simulink model "Controller_bis"  (R2019b)
settings: Solver=VariableStepAuto  StartTime=0.0  StopTime=10.0  RelTol=1e-3
undefined symbols (not defined in the file): B, b1, b2, C, D, gravity, K, KControl, l, q0
settings Model: Creator=ariannagasparri  LastModifiedBy=giga4
settings DebuggingCC: UnderSpecifiedDimensionMsg=warning

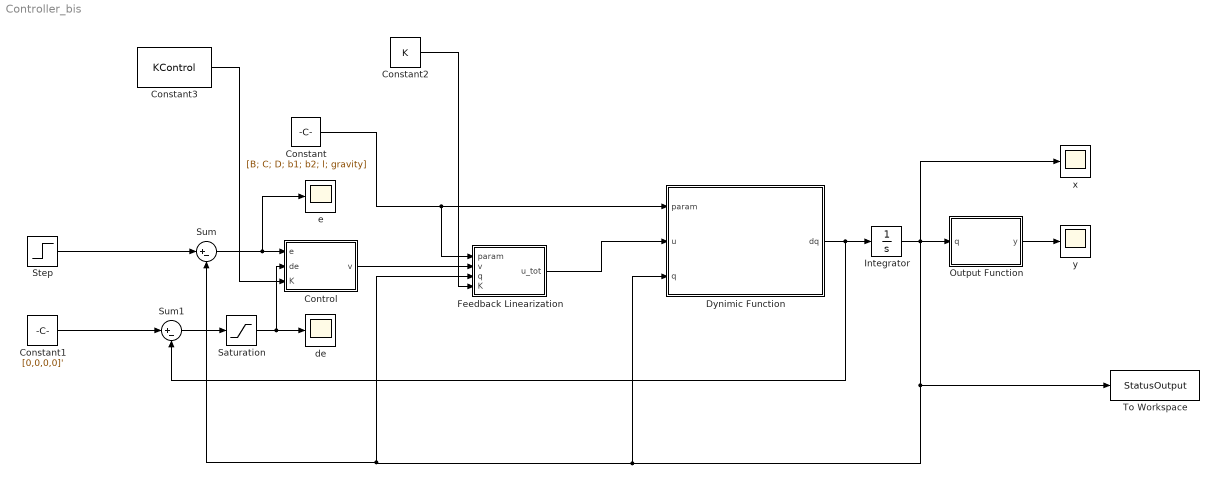
== system Controller_bis ==
  Constant : Constant  Value=[B; C; D; b1; b2; l; gravity]
  Constant1 : Constant  Value=[0,0,0,0]'
  Constant2 : Constant  Value=K
  Constant3 : Constant  Value=KControl
  Control : MATLAB Function  TreatAsAtomicUnit=on
  Dynimic Function : MATLAB Function  TreatAsAtomicUnit=on
  Feedback Linearization : MATLAB Function  TreatAsAtomicUnit=on
  Integrator : Integrator  InitialCondition=q0
  Output Function : MATLAB Function  TreatAsAtomicUnit=on
  Saturation : Saturate  UpperLimit=[10,10,10,10]'  LowerLimit=-[10,10,10,10]'
  Step : Step  After=[0,0,3,0]'  SampleTime=0
  Sum : Sum  Inputs=|+-
  Sum1 : Sum  Inputs=|+-
  To Workspace : ToWorkspace  VariableName=StatusOutput  SaveFormat=Timeseries  SampleTime=-1
  de : Scope
  e : Scope
  x : Scope
  y : Scope
  wires:
  Integrator/1 -> To Workspace/1, Dynimic Function/3(q), Sum/2, Feedback Linearization/3(q), x/1, Output Function/1(q)
  Constant/1 -> Feedback Linearization/1(param), Dynimic Function/1(param)
  Sum1/1 -> Saturation/1
  Dynimic Function/1(dq) -> Sum1/2, Integrator/1
  Sum/1 -> e/1, Control/1(e)
  Output Function/1(y) -> y/1
  Control/1(v) -> Feedback Linearization/2(v)
  Step/1 -> Sum/1
  Constant1/1 -> Sum1/1
  Feedback Linearization/1(u_tot) -> Dynimic Function/2(u)
  Saturation/1 -> Control/2(de), de/1
  Constant2/1 -> Feedback Linearization/4(K)
  Constant3/1 -> Control/3(K)

== matlab function Controller_bis/Feedback Linearization ==
  data: param input; v input; u_tot output; q input; K input
function u_tot = fcn(param, v, q, K)

u = zeros(2,1);

B = param(1);
C = param(2);
D = param(3);
b1 = param(4);
b2 = param(5);
l = param(6);
gravity = param(7);

u(1) = (v(1) - Lf2h1_fun(B,C,D,b1,b2,gravity,l,q)) / LgLfh1_fun(B,C,D,l,q);
u(2) = (v(3) - Lf2h2_fun(B,C,b2,gravity,l,q)) / LgLfh2_fun(B,C,D,l,q);


u_tot = K(1)*u(1) + K(2)*u(2);


end

== matlab function Controller_bis/Dynimic Function ==
  data: param input; u input; dq output; q input
function dq = fcn(param, u, q)

B = param(1);
C = param(2);
D = param(3);
b1 = param(4);
b2 = param(5);
l = param(6);
gravity = param(7);

dq = f_fun(B,C,D,b1,b2,gravity,l,q) + g_fun(B,C,D,l,q)*u;

end

== matlab function Controller_bis/Output Function ==
  data: q input; y output
function y = fcn(q)

y = h_fun(q);

end

== matlab function Controller_bis/Control ==
  data: e input; v output; de input; K input
function v = fcn(e, de, K)

kp = K(1);
kd = K(2);

v = kp * e + kd * de;

end
